simulink model "newnewPMSG"  (R2026a)
settings: Solver=VariableStepAuto  StopTime=0.5
libraries: fl_lib x30, nesl_utility x19, ee_lib x8, simulink x7, slpidlib x6, eeTransforms x4, eePowerMeasurement x1, eeSinusoidalMeasurementV2 x1, mcbeeMathTransformLib x1
(part 2 of 2)

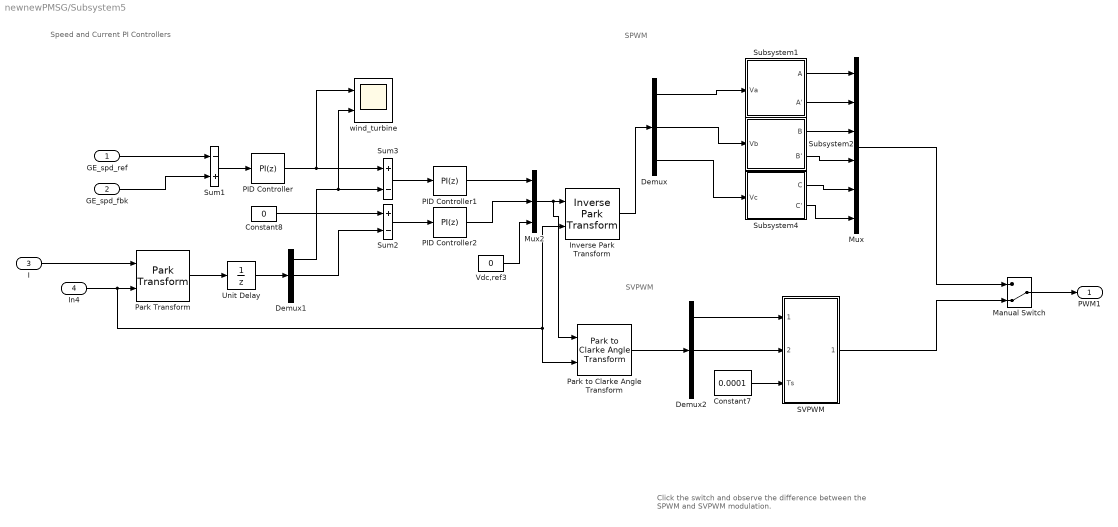
== system newnewPMSG/Subsystem5 ==
  note: Speed and Current PI Controllers
  note: SVPWM
  note: SPWM
  note: Click the switch and observe the difference
      | between the SPWM and SVPWM modulation.
  GE_spd_ref : Inport
  GE_spd_fbk : Inport  Port=2
  I : Inport  Port=3
  In4 : Inport  Port=4
  Constant7 : Constant  Value=0.0001
  Constant8 : Constant  Value=0
  Demux : Demux  Outputs=3
  Demux1 : Demux  Outputs=3
  Demux2 : Demux  Outputs=3
  Inverse Park Transform : eeTransforms/Inverse Park Transform  AxisAlignment=Q-axis  PowerInvariant=off
      settings: LibrarySourceBlock=|
      | ee_sl_lib/Mathematical
      | Transforms/Inverse
      | Park Transform
  Manual Switch : ManualSwitch  CurrentSetting=0
  Mux : Mux  Inputs=6
  Mux2 : Mux  Inputs=3
  PID Controller : slpidlib/PID Controller  Controller=PI  Form=Parallel  TimeDomain=Discrete-time  UseExternalTs=off  SampleTime=-1  IntegratorMethod=Forward Euler  FilterMethod=Forward Euler  ControllerParametersSource=internal  P=100  I=10000  UseKiTs=off  D=0  UseExternalDerivativeSource=off  N=100  UseFilter=on  TunerSelectOption=Transfer Function Based (PID Tuner App)  InitialConditionSource=internal  InitialConditionForIntegrator=0  InitialConditionForFilter=0  DifferentiatorICPrevScaledInput=0  ExternalReset=none  TrackingMode=off  Kt=1  LimitOutput=on  SatLimitsSource=internal  UpperSaturationLimit=1500  LowerSaturationLimit=-1500  LinearizeAsGain=on  AntiWindupMode=none  Kb=1  LimitIntegrator=off  UpperIntegratorSaturationLimit=inf  LowerIntegratorSaturationLimit=-inf  POutMin=[]  POutMax=[]  IOutMin=[]  IOutMax=[]  DOutMin=[]  DOutMax=[]  NOutMin=[]  NOutMax=[]  SumOutMin=[]  SumOutMax=[]  SaturationOutMin=[]  SaturationOutMax=[]  PParamMin=[]  PParamMax=[]  IParamMin=[]  IParamMax=[]  DParamMin=[]  DParamMax=[]  NParamMin=[]  NParamMax=[]  KbParamMin=[]  KbParamMax=[]  KtParamMin=[]  KtParamMax=[]  KbOutMin=[]  KbOutMax=[]  KtOutMin=[]  KtOutMax=[]  IntegratorOutMin=[]  IntegratorOutMax=[]  FilterOutMin=[]  FilterOutMax=[]  SumI1OutMin=[]  SumI1OutMax=[]  SumI2OutMin=[]  SumI2OutMax=[]  SumI3OutMin=[]  SumI3OutMax=[]  SumI4OutMin=[]  SumI4OutMax=[]  SumDOutMin=[]  SumDOutMax=[]  DifferentiatorOutMin=[]  DifferentiatorOutMax=[]  FilterDiffOutCoefMin=[]  FilterDiffOutCoefMax=[]  ReciprocalOutMin=[]  ReciprocalOutMax=[]  SumDenOutMin=[]  SumDenOutMax=[]  SumNumOutMin=[]  SumNumOutMax=[]  DivideOutMin=[]  DivideOutMax=[]  UdiffTsProdOutMin=[]  UdiffTsProdOutMax=[]  NTsProdOutMin=[]  NTsProdOutMax=[]  UintegralTsProdOutMin=[]  UintegralTsProdOutMax=[]  UngainTsProdOutMin=[]  UngainTsProdOutMax=[]  ClampingZeroOutDataTypeStr=Inherit: Inherit via back propagation  ClampingZeroOutMin=[]  ClampingZeroOutMax=[]  FilterDenConstantOutDataTypeStr=Inherit: Inherit via back propagation  FilterDenConstantOutMin=[]  FilterDenConstantOutMax=[]  PCopyOutDataTypeStr=Inherit: Inherit via back propagation  PCopyOutMin=[]  PCopyOutMax=[]  NCopyOutDataTypeStr=Inherit: Inherit via back propagation  NCopyOutMin=[]  NCopyOutMax=[]  IntegratorContinuousStateAttributes=''  IntegratorStateMustResolveToSignalObject=off  IntegratorRTWStateStorageClass=Auto  FilterContinuousStateAttributes=''  FilterStateMustResolveToSignalObject=off  FilterRTWStateStorageClass=Auto  ParallelPVariant=InternalParameters  IdealPVariant=Disabled  IVariant=InternalParameters  DVariant=Disabled  IntegratorVariant=Discrete  SatVariant=Enabled  AWVariant=Passthrough  PCopyVariant=Disabled  TRVariant=Disabled  FdbkBlocksVariant=Forward  IdealPFdbkVariant=Disabled  SatFdbkVariant=Disabled  DerivativeFilterVariant=Disabled  NVariant=Disabled  NCopyVariant=Disabled_SignalSpec  FilterICVariant=Disabled  IntegratorICVariant=InternalICs  ExternalResetVariant=Disabled  TRSumVariant=Passthrough  SumFdbkVariant=Disabled  SumVariant=Sum_PI  TsampFilterVariant=InternalTs  TsampNgainVariant=Passthrough  TsampIntegralVariant=Disabled_SignalSpec  ExternalSaturationOutDataTypeStr=Inherit: Same as second input  DerivativeSourceVariant=Disabled  PreIntVariant=InternalPreInt
  PID Controller1 : slpidlib/PID Controller  Controller=PI  Form=Parallel  TimeDomain=Discrete-time  UseExternalTs=off  SampleTime=-1  IntegratorMethod=Forward Euler  FilterMethod=Forward Euler  ControllerParametersSource=internal  P=1  I=10  UseKiTs=off  D=0  UseExternalDerivativeSource=off  N=100  UseFilter=on  TunerSelectOption=Transfer Function Based (PID Tuner App)  InitialConditionSource=internal  InitialConditionForIntegrator=0  InitialConditionForFilter=0  DifferentiatorICPrevScaledInput=0  ExternalReset=none  TrackingMode=off  Kt=1  LimitOutput=on  SatLimitsSource=internal  UpperSaturationLimit=5  LowerSaturationLimit=-5  LinearizeAsGain=on  AntiWindupMode=none  Kb=1  LimitIntegrator=off  UpperIntegratorSaturationLimit=inf  LowerIntegratorSaturationLimit=-inf  POutMin=[]  POutMax=[]  IOutMin=[]  IOutMax=[]  DOutMin=[]  DOutMax=[]  NOutMin=[]  NOutMax=[]  SumOutMin=[]  SumOutMax=[]  SaturationOutMin=[]  SaturationOutMax=[]  PParamMin=[]  PParamMax=[]  IParamMin=[]  IParamMax=[]  DParamMin=[]  DParamMax=[]  NParamMin=[]  NParamMax=[]  KbParamMin=[]  KbParamMax=[]  KtParamMin=[]  KtParamMax=[]  KbOutMin=[]  KbOutMax=[]  KtOutMin=[]  KtOutMax=[]  IntegratorOutMin=[]  IntegratorOutMax=[]  FilterOutMin=[]  FilterOutMax=[]  SumI1OutMin=[]  SumI1OutMax=[]  SumI2OutMin=[]  SumI2OutMax=[]  SumI3OutMin=[]  SumI3OutMax=[]  SumI4OutMin=[]  SumI4OutMax=[]  SumDOutMin=[]  SumDOutMax=[]  DifferentiatorOutMin=[]  DifferentiatorOutMax=[]  FilterDiffOutCoefMin=[]  FilterDiffOutCoefMax=[]  ReciprocalOutMin=[]  ReciprocalOutMax=[]  SumDenOutMin=[]  SumDenOutMax=[]  SumNumOutMin=[]  SumNumOutMax=[]  DivideOutMin=[]  DivideOutMax=[]  UdiffTsProdOutMin=[]  UdiffTsProdOutMax=[]  NTsProdOutMin=[]  NTsProdOutMax=[]  UintegralTsProdOutMin=[]  UintegralTsProdOutMax=[]  UngainTsProdOutMin=[]  UngainTsProdOutMax=[]  ClampingZeroOutDataTypeStr=Inherit: Inherit via back propagation  ClampingZeroOutMin=[]  ClampingZeroOutMax=[]  FilterDenConstantOutDataTypeStr=Inherit: Inherit via back propagation  FilterDenConstantOutMin=[]  FilterDenConstantOutMax=[]  PCopyOutDataTypeStr=Inherit: Inherit via back propagation  PCopyOutMin=[]  PCopyOutMax=[]  NCopyOutDataTypeStr=Inherit: Inherit via back propagation  NCopyOutMin=[]  NCopyOutMax=[]  IntegratorContinuousStateAttributes=''  IntegratorStateMustResolveToSignalObject=off  IntegratorRTWStateStorageClass=Auto  FilterContinuousStateAttributes=''  FilterStateMustResolveToSignalObject=off  FilterRTWStateStorageClass=Auto  ParallelPVariant=InternalParameters  IdealPVariant=Disabled  IVariant=InternalParameters  DVariant=Disabled  IntegratorVariant=Discrete  SatVariant=Enabled  AWVariant=Passthrough  PCopyVariant=Disabled  TRVariant=Disabled  FdbkBlocksVariant=Forward  IdealPFdbkVariant=Disabled  SatFdbkVariant=Disabled  DerivativeFilterVariant=Disabled  NVariant=Disabled  NCopyVariant=Disabled_SignalSpec  FilterICVariant=Disabled  IntegratorICVariant=InternalICs  ExternalResetVariant=Disabled  TRSumVariant=Passthrough  SumFdbkVariant=Disabled  SumVariant=Sum_PI  TsampFilterVariant=InternalTs  TsampNgainVariant=Passthrough  TsampIntegralVariant=Disabled_SignalSpec  ExternalSaturationOutDataTypeStr=Inherit: Same as second input  DerivativeSourceVariant=Disabled  PreIntVariant=InternalPreInt
  PID Controller2 : slpidlib/PID Controller  Controller=PI  Form=Parallel  TimeDomain=Discrete-time  UseExternalTs=off  SampleTime=-1  IntegratorMethod=Forward Euler  FilterMethod=Forward Euler  ControllerParametersSource=internal  P=1  I=10  UseKiTs=off  D=0  UseExternalDerivativeSource=off  N=100  UseFilter=on  TunerSelectOption=Transfer Function Based (PID Tuner App)  InitialConditionSource=internal  InitialConditionForIntegrator=0  InitialConditionForFilter=0  DifferentiatorICPrevScaledInput=0  ExternalReset=none  TrackingMode=off  Kt=1  LimitOutput=on  SatLimitsSource=internal  UpperSaturationLimit=5  LowerSaturationLimit=-5  LinearizeAsGain=on  AntiWindupMode=none  Kb=1  LimitIntegrator=off  UpperIntegratorSaturationLimit=inf  LowerIntegratorSaturationLimit=-inf  POutMin=[]  POutMax=[]  IOutMin=[]  IOutMax=[]  DOutMin=[]  DOutMax=[]  NOutMin=[]  NOutMax=[]  SumOutMin=[]  SumOutMax=[]  SaturationOutMin=[]  SaturationOutMax=[]  PParamMin=[]  PParamMax=[]  IParamMin=[]  IParamMax=[]  DParamMin=[]  DParamMax=[]  NParamMin=[]  NParamMax=[]  KbParamMin=[]  KbParamMax=[]  KtParamMin=[]  KtParamMax=[]  KbOutMin=[]  KbOutMax=[]  KtOutMin=[]  KtOutMax=[]  IntegratorOutMin=[]  IntegratorOutMax=[]  FilterOutMin=[]  FilterOutMax=[]  SumI1OutMin=[]  SumI1OutMax=[]  SumI2OutMin=[]  SumI2OutMax=[]  SumI3OutMin=[]  SumI3OutMax=[]  SumI4OutMin=[]  SumI4OutMax=[]  SumDOutMin=[]  SumDOutMax=[]  DifferentiatorOutMin=[]  DifferentiatorOutMax=[]  FilterDiffOutCoefMin=[]  FilterDiffOutCoefMax=[]  ReciprocalOutMin=[]  ReciprocalOutMax=[]  SumDenOutMin=[]  SumDenOutMax=[]  SumNumOutMin=[]  SumNumOutMax=[]  DivideOutMin=[]  DivideOutMax=[]  UdiffTsProdOutMin=[]  UdiffTsProdOutMax=[]  NTsProdOutMin=[]  NTsProdOutMax=[]  UintegralTsProdOutMin=[]  UintegralTsProdOutMax=[]  UngainTsProdOutMin=[]  UngainTsProdOutMax=[]  ClampingZeroOutDataTypeStr=Inherit: Inherit via back propagation  ClampingZeroOutMin=[]  ClampingZeroOutMax=[]  FilterDenConstantOutDataTypeStr=Inherit: Inherit via back propagation  FilterDenConstantOutMin=[]  FilterDenConstantOutMax=[]  PCopyOutDataTypeStr=Inherit: Inherit via back propagation  PCopyOutMin=[]  PCopyOutMax=[]  NCopyOutDataTypeStr=Inherit: Inherit via back propagation  NCopyOutMin=[]  NCopyOutMax=[]  IntegratorContinuousStateAttributes=''  IntegratorStateMustResolveToSignalObject=off  IntegratorRTWStateStorageClass=Auto  FilterContinuousStateAttributes=''  FilterStateMustResolveToSignalObject=off  FilterRTWStateStorageClass=Auto  ParallelPVariant=InternalParameters  IdealPVariant=Disabled  IVariant=InternalParameters  DVariant=Disabled  IntegratorVariant=Discrete  SatVariant=Enabled  AWVariant=Passthrough  PCopyVariant=Disabled  TRVariant=Disabled  FdbkBlocksVariant=Forward  IdealPFdbkVariant=Disabled  SatFdbkVariant=Disabled  DerivativeFilterVariant=Disabled  NVariant=Disabled  NCopyVariant=Disabled_SignalSpec  FilterICVariant=Disabled  IntegratorICVariant=InternalICs  ExternalResetVariant=Disabled  TRSumVariant=Passthrough  SumFdbkVariant=Disabled  SumVariant=Sum_PI  TsampFilterVariant=InternalTs  TsampNgainVariant=Passthrough  TsampIntegralVariant=Disabled_SignalSpec  ExternalSaturationOutDataTypeStr=Inherit: Same as second input  DerivativeSourceVariant=Disabled  PreIntVariant=InternalPreInt
  Park Transform : eeTransforms/Park Transform  AxisAlignment=Q-axis  PowerInvariant=off
      settings: LibrarySourceBlock=|
      | ee_sl_lib/Mathematical
      | Transforms/Park Transform
  Park to Clarke Angle Transform : mcbeeMathTransformLib/Park to Clarke Angle Transform  AxisAlignment=Q-axis  UseWithEmbedded=off  PhaseInput=Two inputs  ThetaInput=Sine and Cosine electrical position  AngleInput=Per-unit  N_points=1024
      settings: LibrarySourceBlock=|
      | ee_sl_lib/Mathematical
      | Transforms/Park to Clarke
      | Angle Transform
  SVPWM : Subsystem
  Subsystem1 : Subsystem
  Subsystem2 : Subsystem
  Subsystem4 : Subsystem
  Sum1 : Sum  Inputs=-+
  Sum2 : Sum  Inputs=+-
  Sum3 : Sum  Inputs=+-
  Unit Delay : UnitDelay  SampleTime=-1
  Vdc,ref3 : Constant  Value=0
  wind_turbine : Scope  NumInputPorts=2
      settings: ActiveDisplayYMinimum=-1841.5555  ActiveDisplayYMaximum=1573.99951  DataLoggingVariableName=ScopeData2
  PWM1 : Outport
  wires:
  Sum1/1 -> PID Controller/1
  Sum2/1 -> PID Controller2/1
  Sum3/1 -> PID Controller1/1
  Vdc,ref3/1 -> Mux2/3
  Constant8/1 -> Sum2/1
  Demux1/2 -> Sum2/2
  Demux1/1 -> wind_turbine/2, Sum3/2
  GE_spd_fbk/1 -> Sum1/2
  PID Controller1/1 -> Mux2/1
  PID Controller2/1 -> Mux2/2
  GE_spd_ref/1 -> Sum1/1
  PID Controller/1 -> wind_turbine/1, Sum3/1
  Subsystem1/1(A) -> Mux/1
  Demux/3 -> Subsystem4/1(Vc)
  Subsystem4/1(C) -> Mux/5
  Subsystem4/2(C') -> Mux/6
  Subsystem2/1(B) -> Mux/3
  Subsystem2/2(B') -> Mux/4
  Demux/2 -> Subsystem2/1(Vb)
  Demux/1 -> Subsystem1/1(Va)
  Subsystem1/2(A') -> Mux/2
  Inverse Park Transform/1 -> Demux/1
  I/1 -> Park Transform/1
  Park Transform/1 -> Unit Delay/1
  Mux2/1 -> Inverse Park Transform/1, Park to Clarke Angle Transform/1
  In4/1 -> Park Transform/2, Inverse Park Transform/2, Park to Clarke Angle Transform/2
  Demux2/2 -> SVPWM/2(u-beta)
  Constant7/1 -> SVPWM/3(Ts)
  Demux2/1 -> SVPWM/1(u-alpha)
  Park to Clarke Angle Transform/1 -> Demux2/1
  Mux/1 -> Manual Switch/1
  SVPWM/1(SVPWM) -> Manual Switch/2
  Manual Switch/1 -> PWM1/1
  Unit Delay/1 -> Demux1/1

== system newnewPMSG/V sensor (Three-Phase) ==
  Grounded Neutral (Three-Phase) : ee_lib/Connectors & References/Grounded Neutral (Three-Phase)  port_option=ee.enum.threePhasePort.composite
  PS-Simulink Converter : nesl_utility/PS-Simulink Converter  PhysicalDomain=network_engine_domain  SubClassName=ps_output  LeftPortType=input  RightPortType=output  PseudoPeriodic=off  Frequencies=[]  VectorFormat=inherit  Unit=inherit  AffineConversion=off
  Phase Voltage Sensor (Three-Phase) : ee_lib/Sensors & Transducers/Phase Voltage Sensor (Three-Phase)  port_option=ee.enum.threePhasePort.composite
  ~1 : PMIOPort  Side=Left
  ~2 : PMIOPort  Port=2  Side=Right
  Vabc : Outport
  wires:
  PS-Simulink Converter/1 -> Vabc/1
  connections:
  PS-Simulink Converter/LConn1 -- Phase Voltage Sensor (Three-Phase)/RConn1
  Phase Voltage Sensor (Three-Phase)/LConn1 -- ~1/RConn1 -- ~2/RConn1
  Grounded Neutral (Three-Phase)/LConn1 -- Phase Voltage Sensor (Three-Phase)/RConn2

== system newnewPMSG/voltage sensor ==
  PS-Simulink Converter1 : nesl_utility/PS-Simulink Converter  PhysicalDomain=network_engine_domain  SubClassName=ps_output  LeftPortType=input  RightPortType=output  PseudoPeriodic=off  Frequencies=[]  VectorFormat=inherit  Unit=inherit  AffineConversion=off
  Unit Delay1 : UnitDelay  SampleTime=-1
  Voltage Sensor : fl_lib/Electrical/Electrical Sensors/Voltage Sensor
  + : PMIOPort  Side=Left
  - : PMIOPort  Port=2  Side=Right
  v : Outport
  wires:
  PS-Simulink Converter1/1 -> Unit Delay1/1
  Unit Delay1/1 -> v/1
  connections:
  Voltage Sensor/LConn1 -- +/RConn1
  PS-Simulink Converter1/LConn1 -- Voltage Sensor/RConn1
  Voltage Sensor/RConn2 -- -/RConn1

== system newnewPMSG/Grid Side/S1 ==
  g : Inport
  Diode : fl_lib/Electrical/Electrical Elements/Diode  Vf=1e-3 V  Ron=1e-3 Ohm  Goff=1e-5 1/Ohm  i_specify=off  i_priority=None  i=0 A  i_nominal_specify=off  i_nominal_value=1  i_nominal_unit=A  v_specify=off  v_priority=None  v=0 V  v_nominal_specify=off  v_nominal_value=1  v_nominal_unit=V
  S1 : fl_lib/Electrical/Electrical Elements/Switch  R_closed=1e-3 Ohm  G_open=1e-5 1/Ohm  Threshold=0.5  i_specify=off  i_priority=None  i=0 A  i_nominal_specify=off  i_nominal_value=1  i_nominal_unit=A  v_specify=off  v_priority=None  v=0 V  v_nominal_specify=off  v_nominal_value=1  v_nominal_unit=V
  Simulink-PS Converter : nesl_utility/Simulink-PS Converter  PhysicalDomain=network_engine_domain  SubClassName=ps_input  LeftPortType=input  RightPortType=output  PseudoPeriodic=off  Frequencies=[]  NoiseDistribution=none  NoiseParameters=[]  Unit=1  AffineConversion=off  FilteringAndDerivatives=zero  SimscapeFilterOrder=1  InputFilterTimeConstant=0.001  UdotUserProvided=0
  + : PMIOPort  Side=Left
  - : PMIOPort  Port=2  Side=Right
  wires:
  g/1 -> Simulink-PS Converter/1
  connections:
  -/RConn1 -- S1/RConn2 -- Diode/LConn1
  +/RConn1 -- S1/LConn1 -- Diode/RConn1
  Simulink-PS Converter/RConn1 -- S1/RConn1

== system newnewPMSG/Grid Side/S2 ==
  g : Inport
  Diode : fl_lib/Electrical/Electrical Elements/Diode  Vf=1e-3 V  Ron=1e-3 Ohm  Goff=1e-5 1/Ohm  i_specify=off  i_priority=None  i=0 A  i_nominal_specify=off  i_nominal_value=1  i_nominal_unit=A  v_specify=off  v_priority=None  v=0 V  v_nominal_specify=off  v_nominal_value=1  v_nominal_unit=V
  S1 : fl_lib/Electrical/Electrical Elements/Switch  R_closed=1e-3 Ohm  G_open=1e-5 1/Ohm  Threshold=0.5  i_specify=off  i_priority=None  i=0 A  i_nominal_specify=off  i_nominal_value=1  i_nominal_unit=A  v_specify=off  v_priority=None  v=0 V  v_nominal_specify=off  v_nominal_value=1  v_nominal_unit=V
  Simulink-PS Converter : nesl_utility/Simulink-PS Converter  PhysicalDomain=network_engine_domain  SubClassName=ps_input  LeftPortType=input  RightPortType=output  PseudoPeriodic=off  Frequencies=[]  NoiseDistribution=none  NoiseParameters=[]  Unit=1  AffineConversion=off  FilteringAndDerivatives=zero  SimscapeFilterOrder=1  InputFilterTimeConstant=0.001  UdotUserProvided=0
  + : PMIOPort  Side=Left
  - : PMIOPort  Port=2  Side=Right
  wires:
  g/1 -> Simulink-PS Converter/1
  connections:
  Simulink-PS Converter/RConn1 -- S1/RConn1
  Diode/RConn1 -- S1/LConn1 -- +/RConn1
  Diode/LConn1 -- S1/RConn2 -- -/RConn1

== system newnewPMSG/Grid Side/S3 ==
  g : Inport
  Diode : fl_lib/Electrical/Electrical Elements/Diode  Vf=1e-3 V  Ron=1e-3 Ohm  Goff=1e-5 1/Ohm  i_specify=off  i_priority=None  i=0 A  i_nominal_specify=off  i_nominal_value=1  i_nominal_unit=A  v_specify=off  v_priority=None  v=0 V  v_nominal_specify=off  v_nominal_value=1  v_nominal_unit=V
  S1 : fl_lib/Electrical/Electrical Elements/Switch  R_closed=1e-3 Ohm  G_open=1e-5 1/Ohm  Threshold=0.5  i_specify=off  i_priority=None  i=0 A  i_nominal_specify=off  i_nominal_value=1  i_nominal_unit=A  v_specify=off  v_priority=None  v=0 V  v_nominal_specify=off  v_nominal_value=1  v_nominal_unit=V
  Simulink-PS Converter : nesl_utility/Simulink-PS Converter  PhysicalDomain=network_engine_domain  SubClassName=ps_input  LeftPortType=input  RightPortType=output  PseudoPeriodic=off  Frequencies=[]  NoiseDistribution=none  NoiseParameters=[]  Unit=1  AffineConversion=off  FilteringAndDerivatives=zero  SimscapeFilterOrder=1  InputFilterTimeConstant=0.001  UdotUserProvided=0
  + : PMIOPort  Side=Left
  - : PMIOPort  Port=2  Side=Right
  wires:
  g/1 -> Simulink-PS Converter/1
  connections:
  -/RConn1 -- S1/RConn2 -- Diode/LConn1
  +/RConn1 -- S1/LConn1 -- Diode/RConn1
  Simulink-PS Converter/RConn1 -- S1/RConn1

== system newnewPMSG/Grid Side/S4 ==
  g : Inport
  Diode : fl_lib/Electrical/Electrical Elements/Diode  Vf=1e-3 V  Ron=1e-3 Ohm  Goff=1e-5 1/Ohm  i_specify=off  i_priority=None  i=0 A  i_nominal_specify=off  i_nominal_value=1  i_nominal_unit=A  v_specify=off  v_priority=None  v=0 V  v_nominal_specify=off  v_nominal_value=1  v_nominal_unit=V
  S1 : fl_lib/Electrical/Electrical Elements/Switch  R_closed=1e-3 Ohm  G_open=1e-5 1/Ohm  Threshold=0.5  i_specify=off  i_priority=None  i=0 A  i_nominal_specify=off  i_nominal_value=1  i_nominal_unit=A  v_specify=off  v_priority=None  v=0 V  v_nominal_specify=off  v_nominal_value=1  v_nominal_unit=V
  Simulink-PS Converter : nesl_utility/Simulink-PS Converter  PhysicalDomain=network_engine_domain  SubClassName=ps_input  LeftPortType=input  RightPortType=output  PseudoPeriodic=off  Frequencies=[]  NoiseDistribution=none  NoiseParameters=[]  Unit=1  AffineConversion=off  FilteringAndDerivatives=zero  SimscapeFilterOrder=1  InputFilterTimeConstant=0.001  UdotUserProvided=0
  + : PMIOPort  Side=Left
  - : PMIOPort  Port=2  Side=Right
  wires:
  g/1 -> Simulink-PS Converter/1
  connections:
  Simulink-PS Converter/RConn1 -- S1/RConn1
  Diode/RConn1 -- S1/LConn1 -- +/RConn1
  Diode/LConn1 -- S1/RConn2 -- -/RConn1

== system newnewPMSG/Grid Side/S5 ==
  g : Inport
  Diode : fl_lib/Electrical/Electrical Elements/Diode  Vf=1e-3 V  Ron=1e-3 Ohm  Goff=1e-5 1/Ohm  i_specify=off  i_priority=None  i=0 A  i_nominal_specify=off  i_nominal_value=1  i_nominal_unit=A  v_specify=off  v_priority=None  v=0 V  v_nominal_specify=off  v_nominal_value=1  v_nominal_unit=V
  S1 : fl_lib/Electrical/Electrical Elements/Switch  R_closed=1e-3 Ohm  G_open=1e-5 1/Ohm  Threshold=0.5  i_specify=off  i_priority=None  i=0 A  i_nominal_specify=off  i_nominal_value=1  i_nominal_unit=A  v_specify=off  v_priority=None  v=0 V  v_nominal_specify=off  v_nominal_value=1  v_nominal_unit=V
  Simulink-PS Converter : nesl_utility/Simulink-PS Converter  PhysicalDomain=network_engine_domain  SubClassName=ps_input  LeftPortType=input  RightPortType=output  PseudoPeriodic=off  Frequencies=[]  NoiseDistribution=none  NoiseParameters=[]  Unit=1  AffineConversion=off  FilteringAndDerivatives=zero  SimscapeFilterOrder=1  InputFilterTimeConstant=0.001  UdotUserProvided=0
  + : PMIOPort  Side=Left
  - : PMIOPort  Port=2  Side=Right
  wires:
  g/1 -> Simulink-PS Converter/1
  connections:
  -/RConn1 -- S1/RConn2 -- Diode/LConn1
  +/RConn1 -- S1/LConn1 -- Diode/RConn1
  Simulink-PS Converter/RConn1 -- S1/RConn1

== system newnewPMSG/Grid Side/S6 ==
  g : Inport
  Diode : fl_lib/Electrical/Electrical Elements/Diode  Vf=1e-3 V  Ron=1e-3 Ohm  Goff=1e-5 1/Ohm  i_specify=off  i_priority=None  i=0 A  i_nominal_specify=off  i_nominal_value=1  i_nominal_unit=A  v_specify=off  v_priority=None  v=0 V  v_nominal_specify=off  v_nominal_value=1  v_nominal_unit=V
  S1 : fl_lib/Electrical/Electrical Elements/Switch  R_closed=1e-3 Ohm  G_open=1e-5 1/Ohm  Threshold=0.5  i_specify=off  i_priority=None  i=0 A  i_nominal_specify=off  i_nominal_value=1  i_nominal_unit=A  v_specify=off  v_priority=None  v=0 V  v_nominal_specify=off  v_nominal_value=1  v_nominal_unit=V
  Simulink-PS Converter : nesl_utility/Simulink-PS Converter  PhysicalDomain=network_engine_domain  SubClassName=ps_input  LeftPortType=input  RightPortType=output  PseudoPeriodic=off  Frequencies=[]  NoiseDistribution=none  NoiseParameters=[]  Unit=1  AffineConversion=off  FilteringAndDerivatives=zero  SimscapeFilterOrder=1  InputFilterTimeConstant=0.001  UdotUserProvided=0
  + : PMIOPort  Side=Left
  - : PMIOPort  Port=2  Side=Right
  wires:
  g/1 -> Simulink-PS Converter/1
  connections:
  Simulink-PS Converter/RConn1 -- S1/RConn1
  Diode/RConn1 -- S1/LConn1 -- +/RConn1
  Diode/LConn1 -- S1/RConn2 -- -/RConn1

== system newnewPMSG/Machine Side/S1 ==
  g : Inport
  Diode : fl_lib/Electrical/Electrical Elements/Diode  Vf=1e-3 V  Ron=1e-3 Ohm  Goff=1e-5 1/Ohm  i_specify=off  i_priority=None  i=0 A  i_nominal_specify=off  i_nominal_value=1  i_nominal_unit=A  v_specify=off  v_priority=None  v=0 V  v_nominal_specify=off  v_nominal_value=1  v_nominal_unit=V
  S1 : fl_lib/Electrical/Electrical Elements/Switch  R_closed=1e-3 Ohm  G_open=1e-5 1/Ohm  Threshold=0.5  i_specify=off  i_priority=None  i=0 A  i_nominal_specify=off  i_nominal_value=1  i_nominal_unit=A  v_specify=off  v_priority=None  v=0 V  v_nominal_specify=off  v_nominal_value=1  v_nominal_unit=V
  Simulink-PS Converter : nesl_utility/Simulink-PS Converter  PhysicalDomain=network_engine_domain  SubClassName=ps_input  LeftPortType=input  RightPortType=output  PseudoPeriodic=off  Frequencies=[]  NoiseDistribution=none  NoiseParameters=[]  Unit=1  AffineConversion=off  FilteringAndDerivatives=zero  SimscapeFilterOrder=1  InputFilterTimeConstant=0.001  UdotUserProvided=0
  + : PMIOPort  Side=Left
  - : PMIOPort  Port=2  Side=Right
  wires:
  g/1 -> Simulink-PS Converter/1
  connections:
  Simulink-PS Converter/RConn1 -- S1/RConn1
  S1/LConn1 -- +/RConn1 -- Diode/RConn1
  Diode/LConn1 -- -/RConn1 -- S1/RConn2

== system newnewPMSG/Machine Side/S2 ==
  g : Inport
  Diode : fl_lib/Electrical/Electrical Elements/Diode  Vf=1e-3 V  Ron=1e-3 Ohm  Goff=1e-5 1/Ohm  i_specify=off  i_priority=None  i=0 A  i_nominal_specify=off  i_nominal_value=1  i_nominal_unit=A  v_specify=off  v_priority=None  v=0 V  v_nominal_specify=off  v_nominal_value=1  v_nominal_unit=V
  S1 : fl_lib/Electrical/Electrical Elements/Switch  R_closed=1e-3 Ohm  G_open=1e-5 1/Ohm  Threshold=0.5  i_specify=off  i_priority=None  i=0 A  i_nominal_specify=off  i_nominal_value=1  i_nominal_unit=A  v_specify=off  v_priority=None  v=0 V  v_nominal_specify=off  v_nominal_value=1  v_nominal_unit=V
  Simulink-PS Converter : nesl_utility/Simulink-PS Converter  PhysicalDomain=network_engine_domain  SubClassName=ps_input  LeftPortType=input  RightPortType=output  PseudoPeriodic=off  Frequencies=[]  NoiseDistribution=none  NoiseParameters=[]  Unit=1  AffineConversion=off  FilteringAndDerivatives=zero  SimscapeFilterOrder=1  InputFilterTimeConstant=0.001  UdotUserProvided=0
  + : PMIOPort  Side=Left
  - : PMIOPort  Port=2  Side=Right
  wires:
  g/1 -> Simulink-PS Converter/1
  connections:
  -/RConn1 -- S1/RConn2 -- Diode/LConn1
  +/RConn1 -- S1/LConn1 -- Diode/RConn1
  Simulink-PS Converter/RConn1 -- S1/RConn1

== system newnewPMSG/Machine Side/S3 ==
  g : Inport
  Diode : fl_lib/Electrical/Electrical Elements/Diode  Vf=1e-3 V  Ron=1e-3 Ohm  Goff=1e-5 1/Ohm  i_specify=off  i_priority=None  i=0 A  i_nominal_specify=off  i_nominal_value=1  i_nominal_unit=A  v_specify=off  v_priority=None  v=0 V  v_nominal_specify=off  v_nominal_value=1  v_nominal_unit=V
  S1 : fl_lib/Electrical/Electrical Elements/Switch  R_closed=1e-3 Ohm  G_open=1e-5 1/Ohm  Threshold=0.5  i_specify=off  i_priority=None  i=0 A  i_nominal_specify=off  i_nominal_value=1  i_nominal_unit=A  v_specify=off  v_priority=None  v=0 V  v_nominal_specify=off  v_nominal_value=1  v_nominal_unit=V
  Simulink-PS Converter : nesl_utility/Simulink-PS Converter  PhysicalDomain=network_engine_domain  SubClassName=ps_input  LeftPortType=input  RightPortType=output  PseudoPeriodic=off  Frequencies=[]  NoiseDistribution=none  NoiseParameters=[]  Unit=1  AffineConversion=off  FilteringAndDerivatives=zero  SimscapeFilterOrder=1  InputFilterTimeConstant=0.001  UdotUserProvided=0
  + : PMIOPort  Side=Left
  - : PMIOPort  Port=2  Side=Right
  wires:
  g/1 -> Simulink-PS Converter/1
  connections:
  Simulink-PS Converter/RConn1 -- S1/RConn1
  Diode/RConn1 -- S1/LConn1 -- +/RConn1
  Diode/LConn1 -- S1/RConn2 -- -/RConn1

== system newnewPMSG/Machine Side/S4 ==
  g : Inport
  Diode : fl_lib/Electrical/Electrical Elements/Diode  Vf=1e-3 V  Ron=1e-3 Ohm  Goff=1e-5 1/Ohm  i_specify=off  i_priority=None  i=0 A  i_nominal_specify=off  i_nominal_value=1  i_nominal_unit=A  v_specify=off  v_priority=None  v=0 V  v_nominal_specify=off  v_nominal_value=1  v_nominal_unit=V
  S1 : fl_lib/Electrical/Electrical Elements/Switch  R_closed=1e-3 Ohm  G_open=1e-5 1/Ohm  Threshold=0.5  i_specify=off  i_priority=None  i=0 A  i_nominal_specify=off  i_nominal_value=1  i_nominal_unit=A  v_specify=off  v_priority=None  v=0 V  v_nominal_specify=off  v_nominal_value=1  v_nominal_unit=V
  Simulink-PS Converter : nesl_utility/Simulink-PS Converter  PhysicalDomain=network_engine_domain  SubClassName=ps_input  LeftPortType=input  RightPortType=output  PseudoPeriodic=off  Frequencies=[]  NoiseDistribution=none  NoiseParameters=[]  Unit=1  AffineConversion=off  FilteringAndDerivatives=zero  SimscapeFilterOrder=1  InputFilterTimeConstant=0.001  UdotUserProvided=0
  + : PMIOPort  Side=Left
  - : PMIOPort  Port=2  Side=Right
  wires:
  g/1 -> Simulink-PS Converter/1
  connections:
  -/RConn1 -- S1/RConn2 -- Diode/LConn1
  +/RConn1 -- S1/LConn1 -- Diode/RConn1
  Simulink-PS Converter/RConn1 -- S1/RConn1

== system newnewPMSG/Machine Side/S5 ==
  g : Inport
  Diode : fl_lib/Electrical/Electrical Elements/Diode  Vf=1e-3 V  Ron=1e-3 Ohm  Goff=1e-5 1/Ohm  i_specify=off  i_priority=None  i=0 A  i_nominal_specify=off  i_nominal_value=1  i_nominal_unit=A  v_specify=off  v_priority=None  v=0 V  v_nominal_specify=off  v_nominal_value=1  v_nominal_unit=V
  S1 : fl_lib/Electrical/Electrical Elements/Switch  R_closed=1e-3 Ohm  G_open=1e-5 1/Ohm  Threshold=0.5  i_specify=off  i_priority=None  i=0 A  i_nominal_specify=off  i_nominal_value=1  i_nominal_unit=A  v_specify=off  v_priority=None  v=0 V  v_nominal_specify=off  v_nominal_value=1  v_nominal_unit=V
  Simulink-PS Converter : nesl_utility/Simulink-PS Converter  PhysicalDomain=network_engine_domain  SubClassName=ps_input  LeftPortType=input  RightPortType=output  PseudoPeriodic=off  Frequencies=[]  NoiseDistribution=none  NoiseParameters=[]  Unit=1  AffineConversion=off  FilteringAndDerivatives=zero  SimscapeFilterOrder=1  InputFilterTimeConstant=0.001  UdotUserProvided=0
  + : PMIOPort  Side=Left
  - : PMIOPort  Port=2  Side=Right
  wires:
  g/1 -> Simulink-PS Converter/1
  connections:
  Simulink-PS Converter/RConn1 -- S1/RConn1
  Diode/RConn1 -- S1/LConn1 -- +/RConn1
  Diode/LConn1 -- S1/RConn2 -- -/RConn1

== system newnewPMSG/Machine Side/S6 ==
  g : Inport
  Diode : fl_lib/Electrical/Electrical Elements/Diode  Vf=1e-3 V  Ron=1e-3 Ohm  Goff=1e-5 1/Ohm  i_specify=off  i_priority=None  i=0 A  i_nominal_specify=off  i_nominal_value=1  i_nominal_unit=A  v_specify=off  v_priority=None  v=0 V  v_nominal_specify=off  v_nominal_value=1  v_nominal_unit=V
  S1 : fl_lib/Electrical/Electrical Elements/Switch  R_closed=1e-3 Ohm  G_open=1e-5 1/Ohm  Threshold=0.5  i_specify=off  i_priority=None  i=0 A  i_nominal_specify=off  i_nominal_value=1  i_nominal_unit=A  v_specify=off  v_priority=None  v=0 V  v_nominal_specify=off  v_nominal_value=1  v_nominal_unit=V
  Simulink-PS Converter : nesl_utility/Simulink-PS Converter  PhysicalDomain=network_engine_domain  SubClassName=ps_input  LeftPortType=input  RightPortType=output  PseudoPeriodic=off  Frequencies=[]  NoiseDistribution=none  NoiseParameters=[]  Unit=1  AffineConversion=off  FilteringAndDerivatives=zero  SimscapeFilterOrder=1  InputFilterTimeConstant=0.001  UdotUserProvided=0
  + : PMIOPort  Side=Left
  - : PMIOPort  Port=2  Side=Right
  wires:
  g/1 -> Simulink-PS Converter/1
  connections:
  -/RConn1 -- S1/RConn2 -- Diode/LConn1
  +/RConn1 -- S1/LConn1 -- Diode/RConn1
  Simulink-PS Converter/RConn1 -- S1/RConn1

== system newnewPMSG/Subsystem1/Subsystem1 ==
  Va : Inport
  Add1 : Sum
  Constant8 : Constant  Value=0.5
  Divide : Product  Inputs=*/
  Logical Operator1 : Logic  Operator=NOT  AllPortsSameDT=off  OutDataTypeStr=boolean
  Relational Operator : RelationalOperator  OutDataTypeStr=boolean  ZeroCross=off  InputSameDT=off
  Repeating Sequence : simulink/Sources/Repeating Sequence  rep_seq_t=[0 1/10000/2 1/10000]  rep_seq_y=[0 1 0]
  Vcomp*2 : Constant  Value=12
  A : Outport
  A' : Outport  Port=2
  wires:
  Va/1 -> Divide/1
  Divide/1 -> Add1/1
  Add1/1 -> Relational Operator/2
  Constant8/1 -> Add1/2
  Repeating Sequence/1 -> Relational Operator/1
  Logical Operator1/1 -> A/1
  Relational Operator/1 -> A'/1, Logical Operator1/1
  Vcomp*2/1 -> Divide/2

== system newnewPMSG/Subsystem1/Subsystem2 ==
  Vb : Inport
  Add1 : Sum
  Constant8 : Constant  Value=0.5
  Divide : Product  Inputs=*/
  Logical Operator1 : Logic  Operator=NOT  AllPortsSameDT=off  OutDataTypeStr=boolean
  Relational Operator : RelationalOperator  OutDataTypeStr=boolean  ZeroCross=off  InputSameDT=off
  Repeating Sequence : simulink/Sources/Repeating Sequence  rep_seq_t=[0 1/10000/2 1/10000]  rep_seq_y=[0 1 0]
  Scope1 : Scope  NumInputPorts=2
      settings: ActiveDisplayYMinimum=-0.125  ActiveDisplayYMaximum=1.125  DataLoggingVariableName=ScopeData3
  Scope4 : Scope  NumInputPorts=2
      settings: ActiveDisplayYMinimum=-500  ActiveDisplayYMaximum=500  DataLoggingVariableName=ScopeData3
  Vcomp*2 : Constant  Value=12
  B : Outport
  B' : Outport  Port=2
  wires:
  Vb/1 -> Divide/1
  Divide/1 -> Add1/1
  Add1/1 -> Relational Operator/2, Scope4/2
  Constant8/1 -> Add1/2
  Repeating Sequence/1 -> Scope1/1, Relational Operator/1
  Logical Operator1/1 -> B/1
  Relational Operator/1 -> B'/1, Logical Operator1/1
  Vcomp*2/1 -> Divide/2

== system newnewPMSG/Subsystem1/Subsystem4 ==
  Vc : Inport
  Add1 : Sum
  Constant8 : Constant  Value=0.5
  Divide : Product  Inputs=*/
  Logical Operator1 : Logic  Operator=NOT  AllPortsSameDT=off  OutDataTypeStr=boolean
  Relational Operator : RelationalOperator  OutDataTypeStr=boolean  ZeroCross=off  InputSameDT=off
  Repeating Sequence : simulink/Sources/Repeating Sequence  rep_seq_t=[0 1/10000/2 1/10000]  rep_seq_y=[0 1 0]
  Scope1 : Scope  NumInputPorts=2
      settings: ActiveDisplayYMinimum=-0.125  ActiveDisplayYMaximum=1.125  DataLoggingVariableName=ScopeData3
  Scope4 : Scope  NumInputPorts=2
      settings: ActiveDisplayYMinimum=-500  ActiveDisplayYMaximum=500  DataLoggingVariableName=ScopeData3
  Vcomp*2 : Constant  Value=12
  C : Outport
  C' : Outport  Port=2
  wires:
  Vc/1 -> Divide/1
  Divide/1 -> Add1/1
  Add1/1 -> Relational Operator/2, Scope4/2
  Constant8/1 -> Add1/2
  Repeating Sequence/1 -> Scope1/1, Relational Operator/1
  Logical Operator1/1 -> C/1
  Relational Operator/1 -> C'/1, Logical Operator1/1
  Vcomp*2/1 -> Divide/2

== system newnewPMSG/Subsystem2/Subsystem2 ==
  lembda : Inport
  beta : Inport  Port=2
  R : Inport  Port=3
  V_wind : Inport  Port=4
  Subsystem : Subsystem  mask{c1=0.5176, c2=116, c3=0.4, c4=5, c5=21, c6=0.0068}
  Subsystem1 : Subsystem
  power grid1 : Scope  NumInputPorts=2
      settings: ActiveDisplayYMinimum=-2.09543  ActiveDisplayYMaximum=-0.09543  DataLoggingVariableName=ScopeData4
  Pm : Outport  VectorParamsAs1DForOutWhenUnconnected=off
  Tm : Outport  Port=2  VectorParamsAs1DForOutWhenUnconnected=off
  wires:
  lembda/1 -> Subsystem1/4(lambda), Subsystem/1(lembda)
  beta/1 -> Subsystem/2(beta)
  R/1 -> Subsystem1/1(R)
  Subsystem1/1(Pm) -> Pm/1
  Subsystem1/2(Tm) -> Tm/1
  V_wind/1 -> Subsystem1/2(V_wind)
  Subsystem/1(Cp) -> power grid1/1, Subsystem1/3(Cp)

== system newnewPMSG/Subsystem5/SVPWM ==
  u-alpha : Inport
  u-beta : Inport  Port=2
  Ts : Inport  Port=3
  Constant : Constant  Value=10
  Subsystem : Subsystem
  Subsystem1 : Subsystem
  TaTbTc : Subsystem
  Tx Ty : Subsystem
  XYZ : Subsystem
  αβ / N : Subsystem
  SVPWM : Outport  VectorParamsAs1DForOutWhenUnconnected=off
  wires:
  u-beta/1 -> αβ / N/1(u-β), XYZ/2(u-β)
  u-alpha/1 -> αβ / N/2(u-α), XYZ/1(u-α)
  Ts/1 -> Tx Ty/5(Ts), TaTbTc/3(Ts), XYZ/3(Ts)
  Constant/1 -> XYZ/4(Udc)
  XYZ/1(X) -> Tx Ty/1(X)
  XYZ/2(Y) -> Tx Ty/2(Y)
  XYZ/3(Z) -> Tx Ty/3(Z)
  αβ / N/1(N) -> Tx Ty/4(N), Subsystem/4(N)
  Tx Ty/1(Tx) -> TaTbTc/1(Tx)
  Tx Ty/2(Ty) -> TaTbTc/2(Ty)
  TaTbTc/1(Ta) -> Subsystem/1(Ta)
  TaTbTc/2(Tb) -> Subsystem/2(Tb)
  TaTbTc/3(Tc) -> Subsystem/3(Tc)
  Subsystem/1(Tcm1) -> Subsystem1/1(Tcm1)
  Subsystem/2(Tcm2) -> Subsystem1/2(Tcm2)
  Subsystem/3(Tcm3) -> Subsystem1/3(Tcm3)
  Subsystem1/1(svpwm) -> SVPWM/1

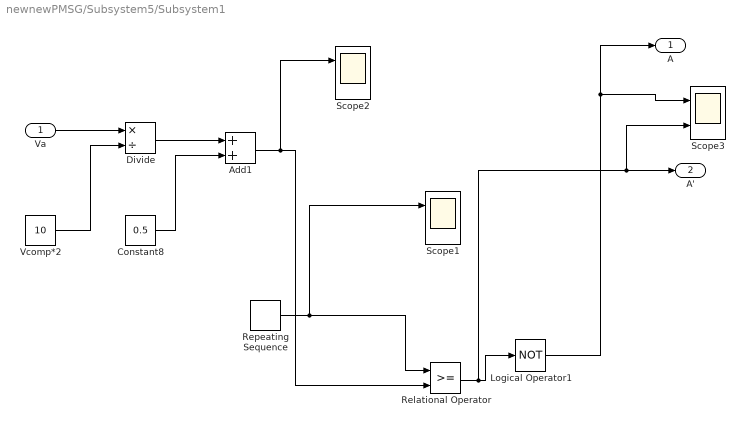
== system newnewPMSG/Subsystem5/Subsystem1 ==
  Va : Inport
  Add1 : Sum
  Constant8 : Constant  Value=0.5
  Divide : Product  Inputs=*/
  Logical Operator1 : Logic  Operator=NOT  AllPortsSameDT=off  OutDataTypeStr=boolean
  Relational Operator : RelationalOperator  OutDataTypeStr=boolean  ZeroCross=off  InputSameDT=off
  Repeating Sequence : simulink/Sources/Repeating Sequence  rep_seq_t=[0 1/10000/2 1/10000]  rep_seq_y=[0 1 0]
  Scope1 : Scope  NumInputPorts=2
      settings: ActiveDisplayYMinimum=-0.12496  ActiveDisplayYMaximum=1.12466  DataLoggingVariableName=ScopeData3
  Scope2 : Scope  NumInputPorts=2
      settings: ActiveDisplayYMinimum=-0.59999  ActiveDisplayYMaximum=3.15933
  Scope3 : Scope  NumInputPorts=2
      settings: ActiveDisplayYMinimum=-0.125  ActiveDisplayYMaximum=1.125  DataLoggingVariableName=ScopeData2
  Vcomp*2 : Constant  Value=10
  A : Outport
  A' : Outport  Port=2
  wires:
  Va/1 -> Divide/1
  Divide/1 -> Add1/1
  Add1/1 -> Scope2/1, Relational Operator/2
  Constant8/1 -> Add1/2
  Repeating Sequence/1 -> Scope1/1, Relational Operator/1
  Logical Operator1/1 -> Scope3/1, A/1
  Relational Operator/1 -> Scope3/2, A'/1, Logical Operator1/1
  Vcomp*2/1 -> Divide/2

== system newnewPMSG/Subsystem5/Subsystem2 ==
  Vb : Inport
  Add1 : Sum
  Constant8 : Constant  Value=0.5
  Divide : Product  Inputs=*/
  Logical Operator1 : Logic  Operator=NOT  AllPortsSameDT=off  OutDataTypeStr=boolean
  Relational Operator : RelationalOperator  OutDataTypeStr=boolean  ZeroCross=off  InputSameDT=off
  Repeating Sequence : simulink/Sources/Repeating Sequence  rep_seq_t=[0 1/10000/2 1/10000]  rep_seq_y=[0 1 0]
  Scope1 : Scope  NumInputPorts=2
      settings: ActiveDisplayYMinimum=-0.125  ActiveDisplayYMaximum=1.125  DataLoggingVariableName=ScopeData3
  Scope4 : Scope  NumInputPorts=2
      settings: ActiveDisplayYMinimum=-500  ActiveDisplayYMaximum=500  DataLoggingVariableName=ScopeData3
  Vcomp*2 : Constant  Value=10
  B : Outport
  B' : Outport  Port=2
  wires:
  Vb/1 -> Divide/1
  Divide/1 -> Add1/1
  Add1/1 -> Relational Operator/2, Scope4/2
  Constant8/1 -> Add1/2
  Repeating Sequence/1 -> Scope1/1, Relational Operator/1
  Logical Operator1/1 -> B/1
  Relational Operator/1 -> B'/1, Logical Operator1/1
  Vcomp*2/1 -> Divide/2

== system newnewPMSG/Subsystem5/Subsystem4 ==
  Vc : Inport
  Add1 : Sum
  Constant8 : Constant  Value=0.5
  Divide : Product  Inputs=*/
  Logical Operator1 : Logic  Operator=NOT  AllPortsSameDT=off  OutDataTypeStr=boolean
  Relational Operator : RelationalOperator  OutDataTypeStr=boolean  ZeroCross=off  InputSameDT=off
  Repeating Sequence : simulink/Sources/Repeating Sequence  rep_seq_t=[0 1/10000/2 1/10000]  rep_seq_y=[0 1 0]
  Scope1 : Scope  NumInputPorts=2
      settings: ActiveDisplayYMinimum=-0.125  ActiveDisplayYMaximum=1.125  DataLoggingVariableName=ScopeData3
  Scope4 : Scope  NumInputPorts=2
      settings: ActiveDisplayYMinimum=-500  ActiveDisplayYMaximum=500  DataLoggingVariableName=ScopeData3
  Vcomp*2 : Constant  Value=10
  C : Outport
  C' : Outport  Port=2
  wires:
  Vc/1 -> Divide/1
  Divide/1 -> Add1/1
  Add1/1 -> Relational Operator/2, Scope4/2
  Constant8/1 -> Add1/2
  Repeating Sequence/1 -> Scope1/1, Relational Operator/1
  Logical Operator1/1 -> C/1
  Relational Operator/1 -> C'/1, Logical Operator1/1
  Vcomp*2/1 -> Divide/2

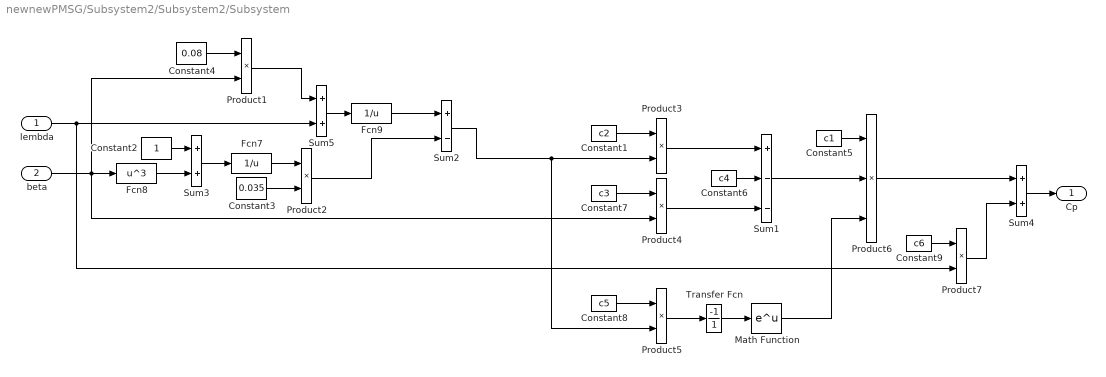
== system newnewPMSG/Subsystem2/Subsystem2/Subsystem ==
  lembda : Inport
  beta : Inport  Port=2
  Constant1 : Constant  Value=c2
  Constant2 : Constant
  Constant3 : Constant  Value=0.035
  Constant4 : Constant  Value=0.08
  Constant5 : Constant  Value=c1
  Constant6 : Constant  Value=c4
  Constant7 : Constant  Value=c3
  Constant8 : Constant  Value=c5
  Constant9 : Constant  Value=c6
  Fcn7 : Fcn  Expr=1/u
  Fcn8 : Fcn  Expr=u^3
  Fcn9 : Fcn  Expr=1/u
  Math Function : Math  SignedPower=on
  Product{1..5,7} (6 alike) : Product  RndMeth=Zero
  Product6 : Product  Inputs=3  RndMeth=Zero
  Sum1 : Sum  Inputs=+--
  Sum2 : Sum  Inputs=+-
  Sum3 : Sum
  Sum4 : Sum
  Sum5 : Sum
  Transfer Fcn : TransferFcn  Numerator=[-1]  Denominator=[1]
  Cp : Outport  VectorParamsAs1DForOutWhenUnconnected=off
  wires:
  Product6/1 -> Sum4/1
  Product7/1 -> Sum4/2
  Constant9/1 -> Product7/1
  Math Function/1 -> Product6/3
  Constant5/1 -> Product6/1
  Sum1/1 -> Product6/2
  Transfer Fcn/1 -> Math Function/1
  Product5/1 -> Transfer Fcn/1
  Constant8/1 -> Product5/1
  Product4/1 -> Sum1/3
  Constant6/1 -> Sum1/2
  Constant7/1 -> Product4/1
  Product3/1 -> Sum1/1
  Constant1/1 -> Product3/1
  Sum2/1 -> Product3/2, Product5/2
  Sum5/1 -> Fcn9/1
  lembda/1 -> Product7/2, Sum5/2
  Product1/1 -> Sum5/1
  Constant4/1 -> Product1/1
  Product2/1 -> Sum2/2
  Constant3/1 -> Product2/2
  Fcn7/1 -> Product2/1
  Fcn8/1 -> Sum3/2
  Sum3/1 -> Fcn7/1
  beta/1 -> Product1/2, Fcn8/1, Product4/2
  Constant2/1 -> Sum3/1
  Fcn9/1 -> Sum2/1
  Sum4/1 -> Cp/1

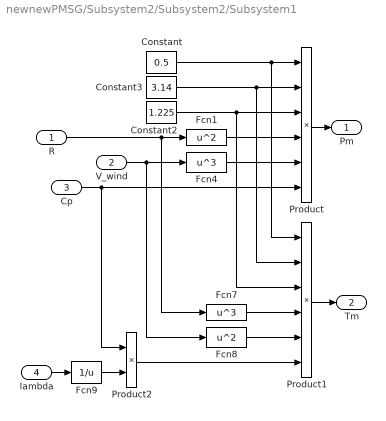
== system newnewPMSG/Subsystem2/Subsystem2/Subsystem1 ==
  R : Inport
  V_wind : Inport  Port=2
  Cp : Inport  Port=3
  lambda : Inport  Port=4
  Constant : Constant  Value=0.5
  Constant2 : Constant  Value=1.225
  Constant3 : Constant  Value=3.14
  Fcn1 : Fcn  Expr=u^2
  Fcn4 : Fcn  Expr=u^3
  Fcn7 : Fcn  Expr=u^3
  Fcn8 : Fcn  Expr=u^2
  Fcn9 : Fcn  Expr=1/u
  Product : Product  Inputs=6  RndMeth=Zero
  Product1 : Product  Inputs=6  RndMeth=Zero
  Product2 : Product  RndMeth=Zero
  Pm : Outport  VectorParamsAs1DForOutWhenUnconnected=off
  Tm : Outport  Port=2  VectorParamsAs1DForOutWhenUnconnected=off
  wires:
  R/1 -> Fcn7/1, Fcn1/1
  V_wind/1 -> Fcn8/1, Fcn4/1
  Constant/1 -> Product/1, Product1/1
  Constant3/1 -> Product/2, Product1/2
  Constant2/1 -> Product/3, Product1/3
  Fcn1/1 -> Product/4
  Fcn4/1 -> Product/5
  Cp/1 -> Product2/1, Product/6
  Fcn7/1 -> Product1/4
  Fcn8/1 -> Product1/5
  Fcn9/1 -> Product2/2
  Product2/1 -> Product1/6
  Product/1 -> Pm/1
  Product1/1 -> Tm/1
  lambda/1 -> Fcn9/1

== system newnewPMSG/Subsystem5/SVPWM/Subsystem ==
  Ta : Inport
  Tb : Inport  Port=2
  Tc : Inport  Port=3
  N : Inport  Port=4
  Multiport Switch : MultiPortSwitch  Inputs=6  SaturateOnIntegerOverflow=off  InputSameDT=off
  Multiport Switch1 : MultiPortSwitch  Inputs=6  SaturateOnIntegerOverflow=off  InputSameDT=off
  Multiport Switch2 : MultiPortSwitch  Inputs=6  SaturateOnIntegerOverflow=off  InputSameDT=off
  Tcm1 : Outport  VectorParamsAs1DForOutWhenUnconnected=off
  Tcm2 : Outport  Port=2  VectorParamsAs1DForOutWhenUnconnected=off
  Tcm3 : Outport  Port=3  VectorParamsAs1DForOutWhenUnconnected=off
  wires:
  N/1 -> Multiport Switch/1, Multiport Switch1/1, Multiport Switch2/1
  Ta/1 -> Multiport Switch2/7, Multiport Switch2/5, Multiport Switch1/6, Multiport Switch1/2, Multiport Switch/4, Multiport Switch/3
  Tb/1 -> Multiport Switch/7, Multiport Switch/2, Multiport Switch1/5, Multiport Switch2/3, Multiport Switch2/6, Multiport Switch1/4
  Tc/1 -> Multiport Switch1/7, Multiport Switch2/2, Multiport Switch2/4, Multiport Switch1/3, Multiport Switch/5, Multiport Switch/6
  Multiport Switch/1 -> Tcm1/1
  Multiport Switch1/1 -> Tcm2/1
  Multiport Switch2/1 -> Tcm3/1

== system newnewPMSG/Subsystem5/SVPWM/Subsystem1 ==
  Tcm1 : Inport
  Tcm2 : Inport  Port=2
  Tcm3 : Inport  Port=3
  Logical Operator : Logic  Operator=NOT  AllPortsSameDT=off  OutDataTypeStr=boolean
  Logical Operator1 : Logic  Operator=NOT  AllPortsSameDT=off  OutDataTypeStr=boolean
  Logical Operator2 : Logic  Operator=NOT  AllPortsSameDT=off  OutDataTypeStr=boolean
  Mux : Mux  Inputs=6
  Relational Operator : RelationalOperator  OutDataTypeStr=boolean  ZeroCross=off  InputSameDT=off
  Relational Operator1 : RelationalOperator  OutDataTypeStr=boolean  ZeroCross=off  InputSameDT=off
  Relational Operator2 : RelationalOperator  OutDataTypeStr=boolean  ZeroCross=off  InputSameDT=off
  Repeating Sequence : simulink/Sources/Repeating Sequence  rep_seq_t=[0 0.00005 0.0001]  rep_seq_y=[0 0.00005 0]
  Scope : Scope
      settings: ActiveDisplayYMinimum=-6E-6  ActiveDisplayYMaximum=5.6E-5  DataLoggingSaveFormat=Array
  svpwm : Outport  VectorParamsAs1DForOutWhenUnconnected=off
  wires:
  Repeating Sequence/1 -> Relational Operator1/1, Relational Operator2/1, Relational Operator/1, Scope/1
  Tcm1/1 -> Relational Operator/2
  Tcm2/1 -> Relational Operator1/2
  Tcm3/1 -> Relational Operator2/2
  Relational Operator/1 -> Logical Operator/1, Mux/1
  Logical Operator/1 -> Mux/2
  Relational Operator1/1 -> Logical Operator1/1, Mux/3
  Logical Operator1/1 -> Mux/4
  Relational Operator2/1 -> Logical Operator2/1, Mux/5
  Logical Operator2/1 -> Mux/6
  Mux/1 -> svpwm/1

== system newnewPMSG/Subsystem5/SVPWM/TaTbTc ==
  Tx : Inport
  Ty : Inport  Port=2
  Ts : Inport  Port=3
  Add : Sum  Inputs=+--
  Add1 : Sum
  Add2 : Sum
  Gain : Gain  Gain=0.5
  Gain1 : Gain  Gain=0.5
  Gain2 : Gain  Gain=0.25
  Ta : Outport  VectorParamsAs1DForOutWhenUnconnected=off
  Tb : Outport  Port=2  VectorParamsAs1DForOutWhenUnconnected=off
  Tc : Outport  Port=3  VectorParamsAs1DForOutWhenUnconnected=off
  wires:
  Ts/1 -> Add/1
  Tx/1 -> Gain/1, Add/2
  Ty/1 -> Gain1/1, Add/3
  Gain/1 -> Add1/2
  Add1/1 -> Add2/1, Tb/1
  Gain1/1 -> Add2/2
  Add2/1 -> Tc/1
  Add/1 -> Gain2/1
  Gain2/1 -> Add1/1, Ta/1

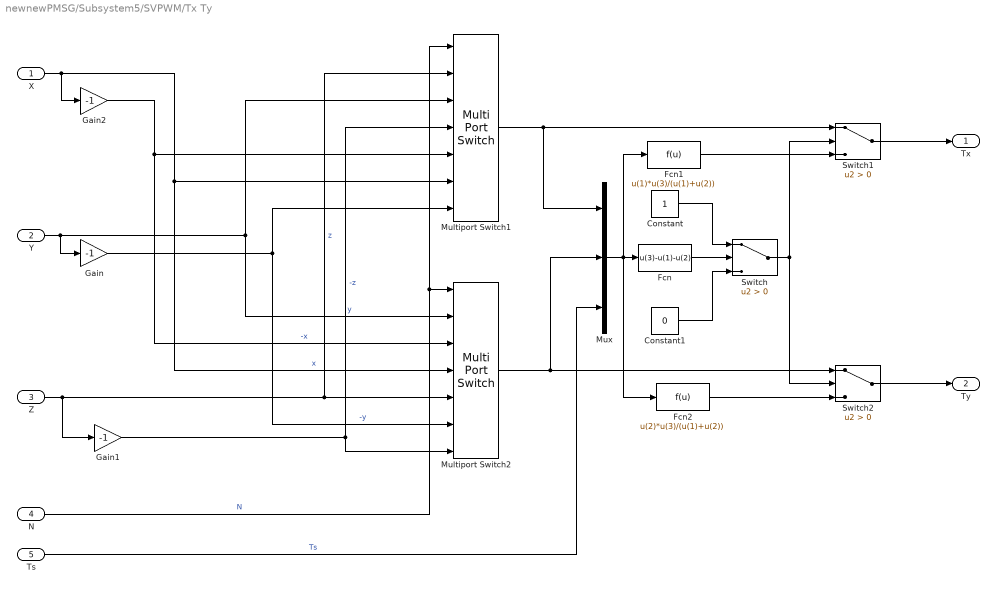
== system newnewPMSG/Subsystem5/SVPWM/Tx Ty ==
  X : Inport
  Y : Inport  Port=2
  Z : Inport  Port=3
  N : Inport  Port=4
  Ts : Inport  Port=5
  Constant : Constant
  Constant1 : Constant  Value=0
  Fcn : Fcn  Expr=u(3)-u(1)-u(2)
  Fcn1 : Fcn  Expr=u(1)*u(3)/(u(1)+u(2))
  Fcn2 : Fcn  Expr=u(2)*u(3)/(u(1)+u(2))
  Gain : Gain  Gain=-1
  Gain1 : Gain  Gain=-1
  Gain2 : Gain  Gain=-1
  Multiport Switch1 : MultiPortSwitch  Inputs=6  SaturateOnIntegerOverflow=off  InputSameDT=off
  Multiport Switch2 : MultiPortSwitch  Inputs=6  SaturateOnIntegerOverflow=off  InputSameDT=off
  Mux : Mux  Inputs=3
  Switch : Switch  Criteria=u2 > Threshold  SaturateOnIntegerOverflow=off  InputSameDT=off
  Switch1 : Switch  Criteria=u2 > Threshold  SaturateOnIntegerOverflow=off  InputSameDT=off
  Switch2 : Switch  Criteria=u2 > Threshold  SaturateOnIntegerOverflow=off  InputSameDT=off
  Tx : Outport  VectorParamsAs1DForOutWhenUnconnected=off
  Ty : Outport  Port=2  VectorParamsAs1DForOutWhenUnconnected=off
  wires:
  N/1 -> Multiport Switch1/1, Multiport Switch2/1  "N"
  Z/1 -> Multiport Switch1/2, Multiport Switch2/5, Gain1/1  "z"
  Y/1 -> Multiport Switch1/3, Multiport Switch2/2, Gain/1  "y"
  Gain/1 -> Multiport Switch1/7, Multiport Switch2/6  "-y"
  Gain1/1 -> Multiport Switch1/4, Multiport Switch2/7  "-z"
  X/1 -> Gain2/1, Multiport Switch1/6, Multiport Switch2/4  "x"
  Gain2/1 -> Multiport Switch1/5, Multiport Switch2/3  "-x"
  Multiport Switch1/1 -> Switch1/1, Mux/1
  Ts/1 -> Mux/3  "Ts"
  Multiport Switch2/1 -> Mux/2, Switch2/1
  Mux/1 -> Fcn2/1, Fcn1/1, Fcn/1
  Fcn/1 -> Switch/2
  Switch/1 -> Switch1/2, Switch2/2
  Switch1/1 -> Tx/1
  Switch2/1 -> Ty/1
  Fcn1/1 -> Switch1/3
  Fcn2/1 -> Switch2/3
  Constant/1 -> Switch/1
  Constant1/1 -> Switch/3

== system newnewPMSG/Subsystem5/SVPWM/XYZ ==
  u-α : Inport
  u-β : Inport  Port=2
  Ts : Inport  Port=3
  Udc : Inport  Port=4
  Fcn : Fcn  Expr=sqrt(3)*u(3)*u(2)/u(4)
  Fcn1 : Fcn  Expr=u(3)*(sqrt(3)*u(2)+3*u(1))/(2*u(4))
  Fcn2 : Fcn  Expr=u(3)*(sqrt(3)*u(2)-3*u(1))/(2*u(4))
  Mux : Mux
  X : Outport  VectorParamsAs1DForOutWhenUnconnected=off
  Y : Outport  Port=2  VectorParamsAs1DForOutWhenUnconnected=off
  Z : Outport  Port=3  VectorParamsAs1DForOutWhenUnconnected=off
  wires:
  u-α/1 -> Mux/1
  u-β/1 -> Mux/2
  Ts/1 -> Mux/3
  Udc/1 -> Mux/4
  Mux/1 -> Fcn2/1, Fcn1/1, Fcn/1
  Fcn/1 -> X/1
  Fcn1/1 -> Y/1
  Fcn2/1 -> Z/1

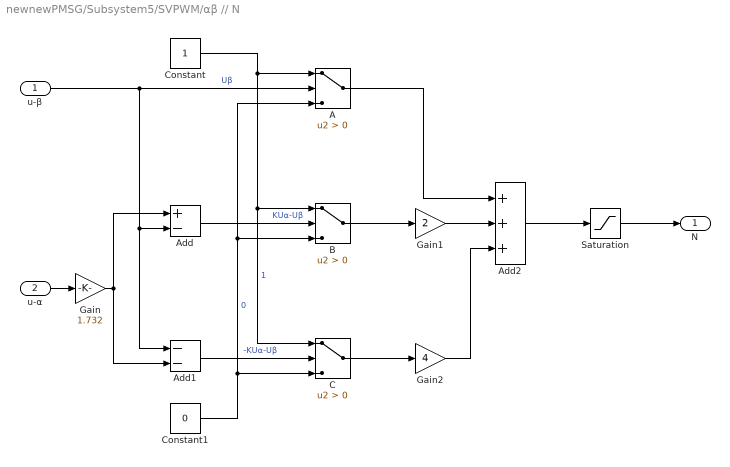
== system newnewPMSG/Subsystem5/SVPWM/αβ // N ==
  u-β : Inport
  u-α : Inport  Port=2
  A : Switch  Criteria=u2 > Threshold  SaturateOnIntegerOverflow=off  InputSameDT=off
  Add : Sum  Inputs=+-
  Add1 : Sum  Inputs=--
  Add2 : Sum  Inputs=+++
  B : Switch  Criteria=u2 > Threshold  SaturateOnIntegerOverflow=off  InputSameDT=off
  C : Switch  Criteria=u2 > Threshold  SaturateOnIntegerOverflow=off  InputSameDT=off
  Constant : Constant
  Constant1 : Constant  Value=0
  Gain : Gain  Gain=1.732
  Gain1 : Gain  Gain=2
  Gain2 : Gain  Gain=4
  Saturation : Saturate  UpperLimit=6  LowerLimit=1
  N : Outport  VectorParamsAs1DForOutWhenUnconnected=off
  wires:
  u-β/1 -> Add1/1, Add/2, A/2  "Uβ"
  Constant/1 -> C/1, B/1, A/1  "1"
  u-α/1 -> Gain/1
  Gain/1 -> Add/1, Add1/2
  Add/1 -> B/2  "KUα-Uβ"
  Constant1/1 -> B/3, A/3, C/3  "0"
  Add1/1 -> C/2  "-KUα-Uβ"
  C/1 -> Gain2/1
  B/1 -> Gain1/1
  A/1 -> Add2/1
  Gain1/1 -> Add2/2
  Gain2/1 -> Add2/3
  Add2/1 -> Saturation/1
  Saturation/1 -> N/1

== matlab function newnewPMSG/electric_angle ==
  data: u input; y output
function y = fcn(u)
    persistent n;
    persistent x;
    if isempty(n)
        n = 0; 
    end
      if isempty(x)
        x = 0; 
      end
    x=u-6.28*n;
    if x >= 6.28
        n = n + 1; 
    end

    y = x;
end
